simulink subsystem "DC"  (R2024a)
settings: Solver=VariableStepAuto  StartTime=0.0  StopTime=inf  RelTol=1e-3
undefined symbols (not defined in the file): DC_dcEnable
settings Model: DefaultTestHarness=EC10x20140x043A0x043E0x043F0x04380x044F_Harness1  Creator=Dell  LastModifiedBy=Dell

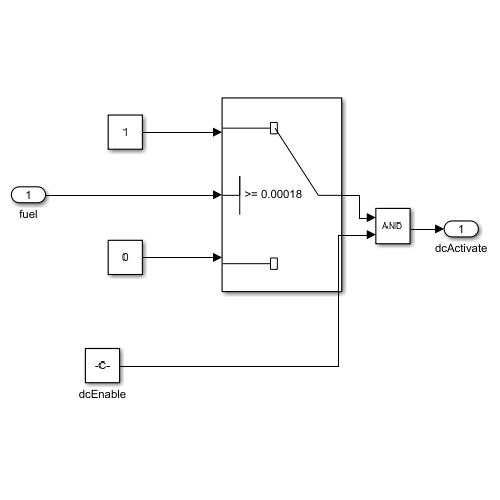
[thumbnail: Simulink's stored preview of the top-level diagram]
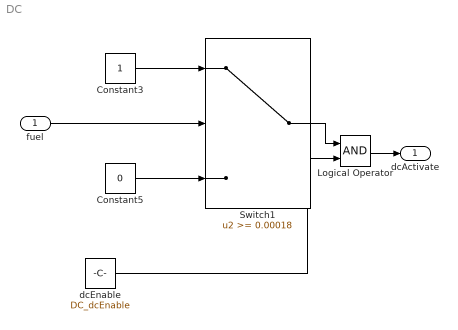
== system DC ==
  fuel : Inport
  Constant3 : Constant
  Constant5 : Constant  Value=0
  Logical Operator : Logic  AllPortsSameDT=off  OutDataTypeStr=boolean
  Switch1 : Switch  Threshold=0.00018  SaturateOnIntegerOverflow=off  InputSameDT=off
  dcEnable : Constant  Value=DC_dcEnable
  dcActivate : Outport
  wires:
  Constant5/1 -> Switch1/3
  Constant3/1 -> Switch1/1
  fuel/1 -> Switch1/2
  Logical Operator/1 -> dcActivate/1
  Switch1/1 -> Logical Operator/1
  dcEnable/1 -> Logical Operator/2
